simulink model "guidance_t3"  (R2019b)
settings: Solver=FixedStepDiscrete  StartTime=0.0  StopTime=inf  FixedStep=0.05  RelTol=1e-3  EnableMultiTasking=on
model workspace (MAT data in the model file):
  SL_ROS_VariableLengthArrays_MaxSizes.CommonInfo.ArrayTruncateAction = 'EmitWarning'
  SL_ROS_VariableLengthArrays_MaxSizes.MsgTypeMap = containers.Map
  SL_ROS_VariableLengthArrays_MaxSizes.MsgTypeMap.serialization.keys = {'sensor_msgs/LaserScan', 'std_msgs/Float64MultiArray'}
  SL_ROS_VariableLengthArrays_MaxSizes.MsgTypeMap.serialization.values{1}(1).PropertyName = 'Intensities'
  SL_ROS_VariableLengthArrays_MaxSizes.MsgTypeMap.serialization.values{1}(1).DataType = 'single'
  SL_ROS_VariableLengthArrays_MaxSizes.MsgTypeMap.serialization.values{1}(1).MaxLength = 360
  SL_ROS_VariableLengthArrays_MaxSizes.MsgTypeMap.serialization.values{1}(2).PropertyName = 'Ranges'
  SL_ROS_VariableLengthArrays_MaxSizes.MsgTypeMap.serialization.values{1}(2).DataType = 'single'
  SL_ROS_VariableLengthArrays_MaxSizes.MsgTypeMap.serialization.values{1}(2).MaxLength = 360
  SL_ROS_VariableLengthArrays_MaxSizes.MsgTypeMap.serialization.values{2}.PropertyName = 'Data'
  SL_ROS_VariableLengthArrays_MaxSizes.MsgTypeMap.serialization.values{2}.DataType = 'double'
  SL_ROS_VariableLengthArrays_MaxSizes.MsgTypeMap.serialization.values{2}.MaxLength = 360
  SL_ROS_VariableLengthArrays_MaxSizes.MsgTypeMap.serialization.uniformity = 0
  SL_ROS_VariableLengthArrays_MaxSizes.MsgTypeMap.serialization.keyType = 'char'
  SL_ROS_VariableLengthArrays_MaxSizes.MsgTypeMap.serialization.valueType = 'any'
undefined symbols (not defined in the file or in its folder): Data, Data_SL_Info, Pose, X, Y, Z
libraries: robotlib x20, sharedtransform x1
settings Model: Creator=USER  LastModifiedBy=nuc
settings DataIOCC: ReturnWorkspaceOutputs=off
settings OptimizationCC: EnhancedBackFolding=on  PassReuseOutputArgsAs=Individual arguments  MaxStackSize=64  OptimizeBlockOrder=speed  DifferentSizesBufferReuse=on  OptimizationCustomize=off  EfficientTunableParamExpr=on
settings DebuggingCC: ParameterTunabilityLossMsg=error  PregeneratedLibrarySubsystemCodeDiagnostic=none  ArithmeticOperatorsInVariantConditions=warning
settings HardwareCC: ProdBitPerPointer=32  ProdBitPerSizeT=32  ProdBitPerPtrDiffT=32  ProdLargestAtomicFloat=None  ProdIntDivRoundTo=Undefined  ProdEndianess=Unspecified  ProdWordSize=32  ProdHWDeviceType=Generic->Unspecified (assume 32-bit Generic)
settings SFSimCC: SimUseLocalCustomCode=off  MATLABDynamicMemAlloc=off  CustomCodeUndefinedFunction=UseInterfaceOnly
settings RTWCC: SystemTargetFile=ert.tlc  HardwareBoard=Robot Operating System (ROS)  TLCOptions="-aInlineSetEventsForThisBaseRateFcn=TLC_FALSE -aSuppressMultiTaskScheduler=TLC_FALSE  -aRateBasedStepFcn=0"  TemplateMakefile=ert_default_tmf  GenerateReport=on  RTWUseLocalCustomCode=off  Toolchain=Catkin  BuildConfiguration=Faster Runs  IncludeHyperlinkInReport=on  LaunchReport=on  TargetLang=C++  GenerateTraceInfo=on  GenerateTraceReport=on  GenerateTraceReportSl=on  GenerateTraceReportSf=on  GenerateTraceReportEml=on
settings CodeAppCC: ForceParamTrailComments=on  IgnoreCustomStorageClasses=off  OperatorAnnotations=on  SimulinkDataObjDesc=on  SFDataObjDesc=on  InsertBlockDesc=on
settings ERTTargetCC: SupportVariableSizeSignals=on

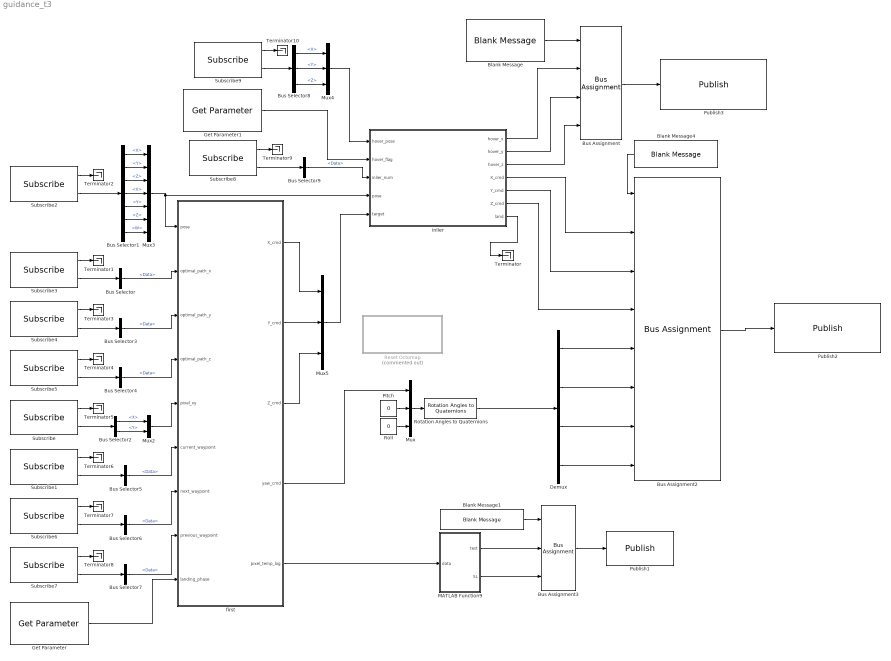
== system guidance_t3 ==
  " Roll" : Constant  Value=0  OutDataTypeStr=double  SampleTime=-1
  Blank Message : robotlib/Blank Message  messageClass=Message  entityType=geometry_msgs/Point  messageType=geometry_msgs/Point  SampleTime=inf
      settings: SourceProductName=ROS Toolbox
  Blank Message1 : robotlib/Blank Message  messageClass=Message  entityType=std_msgs/Float32MultiArray  messageType=std_msgs/Float32MultiArray  SampleTime=-1
      settings: SourceProductBaseCode=RO
  Blank Message4 : robotlib/Blank Message  messageClass=Message  entityType=geometry_msgs/PoseStamped  messageType=geometry_msgs/PoseStamped  SampleTime=-1
      settings: SourceProductBaseCode=RO
  Bus Assignment : BusAssignment  AssignedSignals=X,Y,Z
  Bus Assignment2 : BusAssignment  AssignedSignals=Pose.Position.X,Pose.Position.Y,Pose.Position.Z,Pose.Orientation.W,Pose.Orientation.X,Pose.Orientation.Y,Pose.Orientation.Z
  Bus Assignment3 : BusAssignment  AssignedSignals=Data,Data_SL_Info.CurrentLength
  Bus Selector{,3..7,9} (7 alike) : BusSelector  OutputSignals=Data
  Bus Selector1 : BusSelector  OutputSignals=Pose.Position.X,Pose.Position.Y,Pose.Position.Z,Pose.Orientation.X,Pose.Orientation.Y,Pose.Orientation.Z,Pose.Orientation.W
  Bus Selector2 : BusSelector  OutputSignals=Pose.Position.X,Pose.Position.Y
  Bus Selector8 : BusSelector  OutputSignals=X,Y,Z
  Demux : Demux
  Get Parameter : robotlib/Get Parameter  ParameterSource=Specify your own  ParameterName=/landing_phase  ParameterType=boolean  ParameterMaxArrayLength=16  ParameterInitialValue=false  SampleTime=-1  ShowErrorCodeOutput=off  ModelName=guidance_t2  BlockId=ParamGet_guidance_t2_488
      settings: SourceProductName=ROS Toolbox  SourceProductBaseCode=RR
  Get Parameter1 : robotlib/Get Parameter  ParameterSource=Specify your own  ParameterName=/hover_flag  ParameterType=boolean  ParameterMaxArrayLength=16  ParameterInitialValue=false  SampleTime=-1  ShowErrorCodeOutput=off  ModelName=guidance_t2  BlockId=ParamGet_guidance_t2_489
      settings: SourceProductName=ROS Toolbox  SourceProductBaseCode=RR
  MATLAB Function9 : MATLAB Function  TreatAsAtomicUnit=on
  Mux : Mux  Inputs=3
  Mux2 : Mux  Inputs=2
  Mux3 : Mux  Inputs=7
  Mux4 : Mux  Inputs=3
  Mux5 : Mux  Inputs=3
  Pitch : Constant  Value=0  OutDataTypeStr=double  SampleTime=-1
  Publish1 : robotlib/Publish  topicSource=Specify your own  topic=/pixel_xy_log  messageType=std_msgs/Float32MultiArray  messageQueueLength=1
      settings: SourceProductBaseCode=RO
  Publish2 : robotlib/Publish  topicSource=Select from ROS network  topic=/mavros/setpoint_position/local  messageType=geometry_msgs/PoseStamped  messageQueueLength=1
      settings: SourceProductBaseCode=RO
  Publish3 : robotlib/Publish  topicSource=Specify your own  topic=/hover_pose  messageType=geometry_msgs/Point  messageQueueLength=1
      settings: SourceProductBaseCode=RO
  "Reset Octomap " : Subsystem  Commented=on
  Rotation Angles to Quaternions : sharedtransform/Rotation Angles to Quaternions  rotationOrder=ZYX  aMode=aMode
      settings: SourceProductName=Aerospace Blockset  SourceProductBaseCode=AE
  Subscribe : robotlib/Subscribe  topicSource=Select from ROS network  topic=/pixel_XY  messageType=geometry_msgs/PoseStamped  sampleTime=-1  messageQueueLength=1
      settings: SourceProductBaseCode=RO
  Subscribe1 : robotlib/Subscribe  topicSource=Select from ROS network  topic=/current_point_cmd  messageType=std_msgs/Float32MultiArray  sampleTime=-1  messageQueueLength=1
      settings: SourceProductBaseCode=RO
  Subscribe2 : robotlib/Subscribe  topicSource=Specify your own  topic=/mavros/local_position/pose  messageType=geometry_msgs/PoseStamped  sampleTime=-1  messageQueueLength=1
      settings: SourceProductBaseCode=RO
  Subscribe3 : robotlib/Subscribe  topicSource=Specify your own  topic=/optimal_path_x  messageType=std_msgs/Float32MultiArray  sampleTime=-1  messageQueueLength=1
      settings: SourceProductBaseCode=RO
  Subscribe4 : robotlib/Subscribe  topicSource=Specify your own  topic=/optimal_path_y  messageType=std_msgs/Float32MultiArray  sampleTime=-1  messageQueueLength=1
      settings: SourceProductBaseCode=RO
  Subscribe5 : robotlib/Subscribe  topicSource=Specify your own  topic=/optimal_path_z  messageType=std_msgs/Float32MultiArray  sampleTime=-1  messageQueueLength=1
      settings: SourceProductBaseCode=RO
  Subscribe6 : robotlib/Subscribe  topicSource=Select from ROS network  topic=/next_point_cmd  messageType=std_msgs/Float32MultiArray  sampleTime=-1  messageQueueLength=1
      settings: SourceProductBaseCode=RO
  Subscribe7 : robotlib/Subscribe  topicSource=Select from ROS network  topic=/previous_point_cmd  messageType=std_msgs/Float32MultiArray  sampleTime=-1  messageQueueLength=1
      settings: SourceProductBaseCode=RO
  Subscribe8 : robotlib/Subscribe  topicSource=Specify your own  topic=/rtabmap/inlier_num  messageType=std_msgs/Int16  sampleTime=-1  messageQueueLength=1
      settings: SourceProductBaseCode=RO
  Subscribe9 : robotlib/Subscribe  topicSource=Specify your own  topic=/hover_pose  messageType=geometry_msgs/Point  sampleTime=-1  messageQueueLength=1
      settings: SourceProductBaseCode=RO
  Terminator{,1..10} (11 alike) : Terminator
  first : MATLAB Function  TreatAsAtomicUnit=on
  "inlier " : MATLAB Function  TreatAsAtomicUnit=on
  wires:
  Subscribe2/1 -> Terminator2/1
  Subscribe2/2 -> Bus Selector1/1
  Subscribe3/2 -> Bus Selector/1
  Subscribe3/1 -> Terminator1/1
  Subscribe4/1 -> Terminator3/1
  Subscribe5/1 -> Terminator4/1
  Bus Assignment2/1 -> Publish2/1
  Subscribe4/2 -> Bus Selector3/1
  Subscribe5/2 -> Bus Selector4/1
  Bus Selector/1 -> first/2(optimal_path_x)  "<Data>"
  Bus Selector3/1 -> first/3(optimal_path_y)  "<Data>"
  Bus Selector4/1 -> first/4(optimal_path_z)  "<Data>"
  Bus Selector1/1 -> Mux3/1  "<X>"
  Bus Selector1/2 -> Mux3/2  "<Y>"
  Bus Selector1/3 -> Mux3/3  "<Z>"
  Mux3/1 -> first/1(pose), "inlier "/4(pose)
  Blank Message4/1 -> Bus Assignment2/1
  first/4(yaw_cmd) -> Mux/1
  Mux/1 -> Rotation Angles to Quaternions/1
  Pitch/1 -> Mux/2
  " Roll"/1 -> Mux/3
  Rotation Angles to Quaternions/1 -> Demux/1
  Demux/1 -> Bus Assignment2/5
  Demux/2 -> Bus Assignment2/6
  Demux/3 -> Bus Assignment2/7
  Demux/4 -> Bus Assignment2/8
  Subscribe/1 -> Terminator5/1
  Subscribe/2 -> Bus Selector2/1
  Bus Selector2/1 -> Mux2/1  "<X>"
  Bus Selector2/2 -> Mux2/2  "<Y>"
  Mux2/1 -> first/5(pixel_xy)
  Bus Selector1/6 -> Mux3/6  "<Z>"
  Bus Selector1/7 -> Mux3/7  "<W>"
  MATLAB Function9/2(SL) -> Bus Assignment3/3
  MATLAB Function9/1(test) -> Bus Assignment3/2
  first/5(pixel_temp_log) -> MATLAB Function9/1(data)
  Blank Message1/1 -> Bus Assignment3/1
  Bus Assignment3/1 -> Publish1/1
  first/1(X_cmd) -> Mux5/1
  first/2(Y_cmd) -> Mux5/2
  first/3(Z_cmd) -> Mux5/3
  "inlier "/4(X_cmd) -> Bus Assignment2/2
  "inlier "/5(Y_cmd) -> Bus Assignment2/3
  "inlier "/6(Z_cmd) -> Bus Assignment2/4
  Subscribe1/1 -> Terminator6/1
  Subscribe6/1 -> Terminator7/1
  Subscribe1/2 -> Bus Selector5/1
  Subscribe6/2 -> Bus Selector6/1
  Bus Selector5/1 -> first/6(current_waypoint)  "<Data>"
  Bus Selector6/1 -> first/7(next_waypoint)  "<Data>"
  Subscribe7/1 -> Terminator8/1
  Bus Selector7/1 -> first/8(previous_waypoint)  "<Data>"
  Subscribe7/2 -> Bus Selector7/1
  Bus Selector9/1 -> "inlier "/3(inlier_num)  "<Data>"
  Bus Selector8/1 -> Mux4/1  "<X>"
  Subscribe8/1 -> Terminator9/1
  Mux4/1 -> "inlier "/1(hover_pose)
  Subscribe9/1 -> Terminator10/1
  Subscribe9/2 -> Bus Selector8/1
  Bus Selector8/2 -> Mux4/2  "<Y>"
  Subscribe8/2 -> Bus Selector9/1
  Bus Assignment/1 -> Publish3/1
  Blank Message/1 -> Bus Assignment/1
  Mux5/1 -> "inlier "/5(target)
  "inlier "/1(hover_x) -> Bus Assignment/2
  "inlier "/2(hover_y) -> Bus Assignment/3
  "inlier "/3(hover_z) -> Bus Assignment/4
  Bus Selector1/4 -> Mux3/4  "<X>"
  Bus Selector1/5 -> Mux3/5  "<Y>"
  Bus Selector8/3 -> Mux4/3  "<Z>"
  Get Parameter/1 -> first/9(landing_phase)
  Get Parameter1/1 -> "inlier "/2(hover_flag)
  "inlier "/7(land) -> Terminator/1

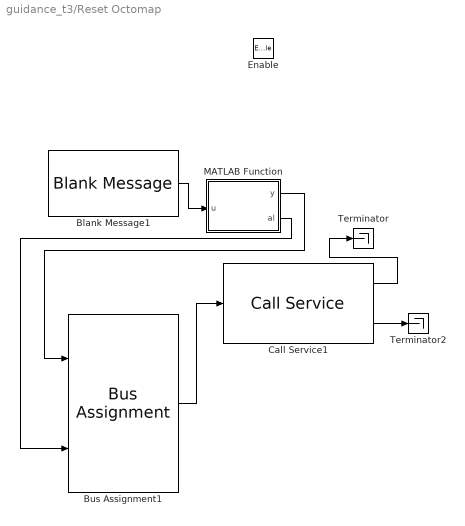
== system guidance_t3/Reset Octomap  ==
  Enable : EnablePort
  Blank Message1 : robotlib/Blank Message  messageClass=Service Request  entityType=mavros/CommandTOL  messageType=mavros/CommandTOLRequest  SampleTime=inf
      settings: SourceProductBaseCode=RO
  Bus Assignment1 : BusAssignment  AssignedSignals=Altitude
  Call Service1 : robotlib/Call Service  topicSource=Specify your own  service=/mavros/cmd/land  serviceType=mavros/CommandTOL  connectionTimeout=5  keepPersistent=off  ShowErrorCodeOutput=on
      settings: SourceProductName=ROS Toolbox  SourceProductBaseCode=RR
  MATLAB Function : MATLAB Function  TreatAsAtomicUnit=on
  Terminator : Terminator
  Terminator2 : Terminator
  wires:
  Bus Assignment1/1 -> Call Service1/1
  MATLAB Function/1(y) -> Bus Assignment1/1
  Blank Message1/1 -> MATLAB Function/1(u)
  Call Service1/1 -> Terminator/1
  Call Service1/2 -> Terminator2/1
  MATLAB Function/2(al) -> Bus Assignment1/2

== matlab function guidance_t3/Reset Octomap /MATLAB Function ==
  data: u input Bus: SL_Bus_guidance_t2_mavros_CommandTOLRequest; y output Bus: SL_Bus_guidance_t2_mavros_CommandTOLRequest; al output
function [y, al]= fcn(u)
    u.Yaw=single(nan);
    u.Latitude = single(nan);
    u.Longitude = single(nan);
    al = single(0);
y = u;

== matlab function guidance_t3/inlier  ==
  data: hover_pose input; hover_flag input; inlier_num input; hover_x output; hover_y output; hover_z output; pose input; X_cmd output; target input; Y_cmd output; Z_cmd output; land output
function [hover_x, hover_y, hover_z, X_cmd, Y_cmd, Z_cmd, land] = fcn(hover_pose, hover_flag, inlier_num, pose, target)
    %% user input
        danger_inlier_num = 10.0;
        danger_hover_enabled = false; 
        danger_move_backward_enabled = false;
        inlier_num_cont_enable = false;
    %% persistent
        persistent XYZ_cmd_temp
        persistent inlier_num_record danger
        persistent hover_pose_saved
        persistent prev_wap prev_wap_temp
    %%
        if isempty(XYZ_cmd_temp)
            XYZ_cmd_temp = [0, 0, 0];
        end
    land = 0;
    if isnan(XYZ_cmd_temp(1)) && sqrt(pose(1)^2 + pose(2)^2) > 0.5
        X_cmd = nan;
        Y_cmd = nan;
        Z_cmd = nan;
        hover_x = nan;
        hover_y = nan;
        hover_z = nan;
    else
        if inlier_num_cont_enable
            %% inlier criteria definition

                    if isempty(inlier_num_record)
                        inlier_num_record = [200, 200, 200, 200, 200, 200, 200, 200, 200, 200];
                    end
                    if isempty(danger)
                        danger = false;
                    end
                inlier_num_current = [double(inlier_num)];
                inlier_num_record = [inlier_num_record([2:end]), inlier_num_current];
                fprintf("inlier num : [%d], avg : [%f]", inlier_num, mean(inlier_num_record, 'all'));
                if mean(inlier_num_record, 'all') < danger_inlier_num
                    fprintf("    Danger !! \n");
                    danger = true;
                else
                    danger = false;
                end

            %% ready_hovor
                    if isempty(hover_pose_saved)
                        hover_pose_saved = false;
                    end
                    if not(hover_pose_saved)
                        hover_x = pose(1);
                        hover_y = pose(2);
                        hover_z = pose(3);
                        hover_pose_saved = true;
                    else
                        hover_x = hover_pose(1);
                        hover_y = hover_pose(2);
                        hover_z = hover_pose(3);
                    end

            %% for ready_move backward
                    if isempty(prev_wap)
                        prev_wap = [0, 0, 0];
                    end
                    if isempty(prev_wap_temp)
                        prev_wap_temp = [0, 0, 0];
                    end

                if (prev_wap_temp(1) ~= target(1)) && (prev_wap_temp(2) ~= target(2)) && (prev_wap_temp(3) ~= target(3))
                    prev_wap(1) = prev_wap_temp(1);
                    prev_wap(2) = prev_wap_temp(2);
                    prev_wap(3) = prev_wap_temp(3);
                end
                    prev_wap_temp(1) = target(1);
                    prev_wap_temp(2) = target(2);
                    prev_wap_temp(3) = target(3);

            %% command
                if danger
                    if danger_hover_enabled
                        fprintf("danger! hovering enabled\n");
                        if hover_pose_saved
                            X_cmd = hover_pose(1);
                            Y_cmd = hover_pose(2);
                            Z_cmd = hover_pose(3);
                        else
                            X_cmd = pose(1);
                            Y_cmd = pose(2);
                            Z_cmd = pose(3);
                        end
                    elseif danger_move_backward_enabled
                        fprintf("danger! move backward enabled\n");
                        X_cmd = pose(1) - (pose(1) - prev_wap(1))/10;
                        Y_cmd = pose(2) - (pose(2) - prev_wap(2))/10;
                        Z_cmd = pose(3) - (pose(3) - prev_wap(3))/10;
                    end
                else
                    if danger_hover_enabled
                        hover_pose_saved = false;
                    end
                    X_cmd = target(1);
                    Y_cmd = target(2);
                    Z_cmd = target(3);
                end
        else
            %% ready_hovor
            if isempty(hover_pose_saved)
                hover_pose_saved = false;
            end
            if not(hover_pose_saved)
                hover_x = pose(1);
                hover_y = pose(2);
                hover_z = pose(3);
                hover_pose_saved = true;
            else
                hover_x = hover_pose(1);
                hover_y = hover_pose(2);
                hover_z = hover_pose(3);
            end
            
            if hover_flag
                X_cmd = hover_x;
                Y_cmd = hover_y;
                Z_cmd = hover_z;
            else
                X_cmd = target(1);
                Y_cmd = target(2);
                Z_cmd = target(3);
            end
        end
    end
    
    if isnan(X_cmd) || isnan(Y_cmd) || isnan(Z_cmd)
        land = 1;
    end
    % ----------------------------------------------------------------------
    % Safety
    % ----------------------------------------------------------------------

    % if pose(1) == 0 && pose(2) == 0 && pose(3) == 0
%     if inlier_num==0
%         Z_cmd = nan(1,1);
%         X_cmd = nan(1,1);
%         Y_cmd = nan(1,1);
%     end
    
    XYZ_cmd_temp = [X_cmd, Y_cmd, Z_cmd];

== matlab function guidance_t3/MATLAB Function9 ==
  data: data input size=[10 1]; test output size=[1 128]; SL output
function [test,SL]   = func(data)

% test = single(nan(1,128));

test = single([data', nan(1,118)]);
% for i = 1:length(data)
%     test(i) = single(data(i));
% end

SL = uint32(length(data));


end

== matlab function guidance_t3/first ==
  data: X_cmd output; Y_cmd output; pose input; Z_cmd output; optimal_path_x input size=[128 1]; optimal_path_y input size=[128 1]; optimal_path_z input size=[128 1]; yaw_cmd output; pixel_xy input; pixel_temp_log output; current_waypoint input; next_waypoint input; previous_waypoint input; landing_phase input
function [X_cmd,Y_cmd,Z_cmd,yaw_cmd,pixel_temp_log] = fcn(pose, optimal_path_x,optimal_path_y,optimal_path_z,pixel_xy,current_waypoint,next_waypoint,previous_waypoint,landing_phase)

persistent yaw_mem yaw_inc hz_20 pixel_temp 
persistent landing_x landing_y landing_hz landing_not_found curr_z_cmd waypoint_changing_phase

goal_point = [-1.6 -3.6 1.2];

if isempty(yaw_mem)
    yaw_mem = 0;
    yaw_inc = 0;
    hz_20 = 0;
    pixel_temp = zeros(5,2);
    waypoint_changing_phase = false;
    
    landing_x = 0;
    landing_y = 0;
    landing_hz = 0;
    landing_not_found = 0;
    curr_z_cmd = goal_point(3);
end

hz_20 = hz_20 + 1;

% ----------------------------------------------------------------------
% Landing
% ----------------------------------------------------------------------

if landing_phase
    pixel_xy = pixel_xy';
    if isempty(pixel_xy)
        pixel_xy = [0,0];
    end

    if landing_hz >= 10
        euler_angle = quat2eul([pose(4),pose(5),pose(6),pose(7)]);
        m = 1.5;
            if landing_x == 0 && landing_y == 0
                landing_x = pose(1)+(m*pixel_xy(2)*cos(euler_angle(1)) + -m*pixel_xy(1)*-sin(euler_angle(1)))*pose(3)/640;
                landing_y = pose(2)+(-m*pixel_xy(1)*cos(euler_angle(1)) + m*pixel_xy(2)*sin(euler_angle(1)))*pose(3)/640;
            else
                if pixel_xy(1) ~= 0 && pixel_xy(2) ~= 0
                    landing_x = (landing_x + pose(1)+(m*pixel_xy(2)*cos(euler_angle(1)) + -m*pixel_xy(1)*-sin(euler_angle(1)))*pose(3)/640)/2;
                    landing_y = (landing_y + pose(2)+(-m*pixel_xy(1)*cos(euler_angle(1)) + m*pixel_xy(2)*sin(euler_angle(1)))*pose(3)/640)/2;
                end
            end
        X_cmd = landing_x;
        Y_cmd = landing_y;
        Z_cmd = -3;
        
        if pose(3) < 0.25
            X_cmd = nan;
            Y_cmd = nan;
            Z_cmd = nan;
        end
    else
        if pixel_xy(1) ~= 0 && pixel_xy(2) ~= 0
            landing_hz = landing_hz + 1;
            X_cmd = goal_point(1);
            Y_cmd = goal_point(2);
            Z_cmd = curr_z_cmd;
        else
            X_cmd = goal_point(1);
            Y_cmd = goal_point(2);
            Z_cmd = goal_point(3);
            if landing_not_found < 300 && landing_not_found >= 150
                X_cmd = goal_point(1);
                Y_cmd = goal_point(2);
                curr_z_cmd = 1.6;
                Z_cmd = curr_z_cmd;
                fprintf("heliport decection failed, z_cmd = 1.6 \n");
            elseif landing_not_found >= 300
                X_cmd = goal_point(1);
                Y_cmd = goal_point(2);
                curr_z_cmd = 2.0;
                Z_cmd = curr_z_cmd;
                fprintf("heliport decection failed, z_cmd = 2.0 \n");
            end
            landing_not_found = landing_not_found + 1;
            if landing_not_found >= 1000
                X_cmd = goal_point(1);
                Y_cmd = goal_point(2);
                Z_cmd = 0;
                fprintf("heliport detection failed \n");
            end
        end 
        fprintf("landing_hz : %f    landing_not_found : %f\n", single(landing_hz), single(landing_not_found));
    end
    yaw_cmd = double(atan2(0,(-1.6)-(5.5)));
else
    % ----------------------------------------------------------------------
    % Traveling
    % ----------------------------------------------------------------------
    
    path_length = length(optimal_path_x);
    K = inf(path_length,1);
    optimal_path_norm = inf(path_length,3);
    
    optimal_path_norm(:,1) = single(optimal_path_x - pose(1));
    optimal_path_norm(:,2) = single(optimal_path_y - pose(2));
    optimal_path_norm(:,3) = single(optimal_path_z - pose(3));
           
    for i=1:path_length
        K(i) = norm(optimal_path_norm(i,:));
    end
    
    [~,m] = min(K);
    
    if m >= 128
        m = 127;
    end

    Z_cmd = double(optimal_path_z(m+1));         % prediction
    X_cmd = double(optimal_path_x(m+1));
    Y_cmd = double(optimal_path_y(m+1));
    
    if m <= 125
        yaw_vector1 = [optimal_path_x(m+1)-pose(1) optimal_path_y(m+1)-pose(2)];
        yaw_vector2 = [optimal_path_x(m+2)-pose(1) optimal_path_y(m+2)-pose(2)];
        yaw_vector3 = [optimal_path_x(m+3)-pose(1) optimal_path_y(m+3)-pose(2)];
        yaw_vector = yaw_vector1 + yaw_vector2 + yaw_vector3;
        if norm(yaw_vector3) <= 0.4
            yaw_cmd = 0;
        else
            yaw_cmd = double( atan2(yaw_vector(2),yaw_vector(1)) );
        end
        yaw_mem = yaw_cmd;
        yaw_inc = 0;
    else
        yaw_cmd = yaw_mem + deg2rad(yaw_inc);
    end
    
    if hz_20 == 80
        hz_20 = 0;
        if m == 128
            yaw_inc = yaw_inc + 30;        % 4초마다 30도 돌려서 관찰
        end
    end

 % ----------------------------------------------------------------------
 % Yaw command at changing waypoint
 % ----------------------------------------------------------------------
    if sqrt((pose(1)-current_waypoint(1))^2+(pose(2)-current_waypoint(2))^2)<0.8
        yaw_cmd = double(atan2(next_waypoint(2)-current_waypoint(2),next_waypoint(1)-current_waypoint(1)));
        waypoint_changing_phase = true;
    end
    if sqrt((pose(1)-previous_waypoint(1))^2+(pose(2)-previous_waypoint(2))^2)<0.8
        yaw_cmd = double(atan2(current_waypoint(2)-previous_waypoint(2),current_waypoint(1)-previous_waypoint(1)));
    end
end
pixel_temp_log = [pixel_temp(:,1);pixel_temp(:,2)];

end
